simulink model "OpAmpOpenLoop"  (R2021b)
settings: Solver=VariableStepAuto  StartTime=0.0  StopTime=inf  MaxStep=1e-4  RelTol=1e-3
libraries: fl_lib x6, nesl_utility x4, ee_lib x1
settings Model: PacingRate=0.010000  Creator=Work  LastModifiedBy=Work

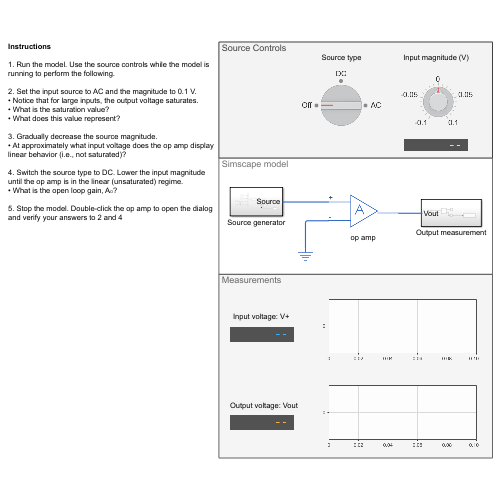
[thumbnail: Simulink's stored preview of the top-level diagram]
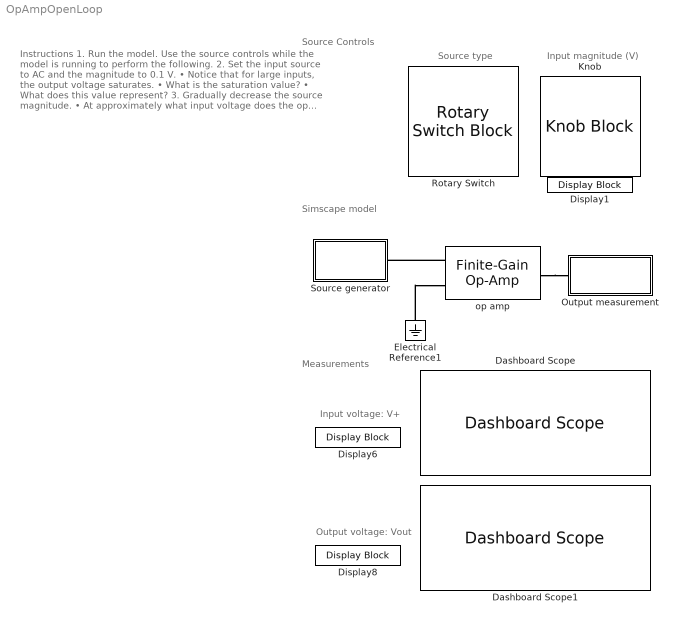
== system OpAmpOpenLoop ==
  note: Input magnitude (V)
  note: Source type
  note: Instructions
      |
      | 1. Run the model. Use the source controls while the model is running to perform the following.
      |
      | 2. Set the input source to AC and the magnitude to 0.1 V.
      | • Notice that for large inputs, the output voltage saturates.
      | • What is the saturation value?
      | • What does this value represent?
      |
      | 3. Gradually decrease the source magnitude.
      | • At approximately what input voltage does the op amp display linear behavior (i.e., not saturated)?
      |
      | 4. Switch the source type to DC. Lower the input magnitude until the op amp is in the linear (unsaturated) regime.
      | • What is the open loop gain, A O ?
      |
      | 5. Stop the model. Double-click the op amp to open the dialog and verify your answers to 2 and 4
  note: Source Controls
  note: Measurements
  note: Simscape model
  note: Input voltage: V+
  note: Output voltage: Vout
  Dashboard Scope : DashboardScope  TimeSpan=0.10000000000000001  Ymin=-0.15  Ymax=0.15  ScaleAtStop=off  UpdateMode=Scroll
  Dashboard Scope1 : DashboardScope  TimeSpan=0.10000000000000001  Ymin=-16  Ymax=16  ScaleAtStop=off  UpdateMode=Scroll
  Display1 : DisplayBlock  LabelPosition=Hide  Format=Custom  Alignment=Right  Transparency=1  FormatString=%0.4f
  Display6 : DisplayBlock  LabelPosition=Hide  Format=Custom  Alignment=Right  Transparency=1  FormatString=%0.4f
  Display8 : DisplayBlock  LabelPosition=Hide  Format=Custom  Alignment=Right  Transparency=1  FormatString=%0.4f
  Electrical Reference1 : fl_lib/Electrical/Electrical Elements/Electrical Reference
  Knob : KnobBlock  LabelPosition=Hide  ScaleMin=-0.1  ScaleMax=0.1  TickInterval=0.05
  Output measurement : Subsystem
  Rotary Switch : RotarySwitchBlock  LabelPosition=Hide
      settings: Values={{'Off', 'DC', 'AC'}, [0 1 2]}
  Source generator : Subsystem
  op amp : ee_lib/Integrated Circuits/Finite-Gain Op-Amp  A=2e3  Rin=1e6 Ohm  Rout=100 Ohm  Vmin=-15 V  Vmax=15 V  noise_mode=0  v_noise=30e-9 V/Hz^(1/2)  noise_prm=1  i_noise=0.5e-12 A/Hz^(1/2)  ip_noise=0.5e-12 A/Hz^(1/2)  in_noise=0.5e-12 A/Hz^(1/2)  sample_time=1e-3 s  repeatability=1  auto_seed_v=1041471841  auto_seed_ip=230873357  auto_seed_in=1897181789  user_seed_v=0  user_seed_ip=0  user_seed_in=0
      settings: SourceProductBaseCode=PS  InternalSimscapePortConfiguration="{\"Bottom\":[],\"Left\":[{\"id\":\"p\",\"label\":\"+\",\"type\":\"foundation.electrical.electrical\"},{\"id\":\"n\",\"label\":\"-\",\"type\":\"foundation.electrical.electrical\"}],\"Right\":[{\"id\":\"out\",\"label\":\"\",\"type\":\"foundation.electrical.electrical\"}],\"Top\":[]}"
  connections:
  Electrical Reference1/LConn1 -- op amp/LConn2
  op amp/LConn1 -- Source generator/RConn1
  op amp/RConn1 -- Output measurement/LConn1

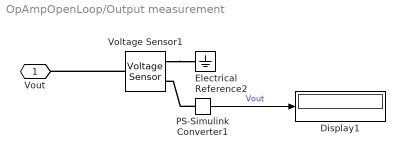
== system OpAmpOpenLoop/Output measurement ==
  Display1 : Display
  Electrical Reference2 : fl_lib/Electrical/Electrical Elements/Electrical Reference
  PS-Simulink Converter1 : nesl_utility/PS-Simulink Converter  PhysicalDomain=network_engine_domain  SubClassName=ps_output  LeftPortType=input  RightPortType=output  PseudoPeriodic=off  Frequencies=[]  Unit=inherit  AffineConversion=off
      settings: SourceProductBaseCode=PW,SS
  Voltage Sensor1 : fl_lib/Electrical/Electrical Sensors/Voltage Sensor
  Vout : PMIOPort  Side=Left
  wires:
  PS-Simulink Converter1/1 -> Display1/1  "Vout"
  connections:
  Voltage Sensor1/LConn1 -- Vout/RConn1
  Voltage Sensor1/RConn2 -- Electrical Reference2/LConn1
  PS-Simulink Converter1/LConn1 -- Voltage Sensor1/RConn1

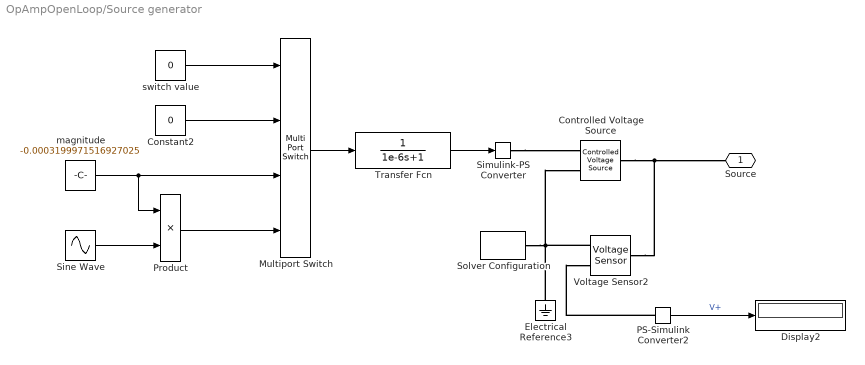
== system OpAmpOpenLoop/Source generator ==
  Constant2 : Constant  Value=0
  Controlled Voltage Source : fl_lib/Electrical/Electrical Sources/Controlled Voltage Source
  Display2 : Display
  Electrical Reference3 : fl_lib/Electrical/Electrical Elements/Electrical Reference
  Multiport Switch : MultiPortSwitch  DataPortOrder=Zero-based contiguous  zeroidx=on
  PS-Simulink Converter2 : nesl_utility/PS-Simulink Converter  PhysicalDomain=network_engine_domain  SubClassName=ps_output  LeftPortType=input  RightPortType=output  PseudoPeriodic=off  Frequencies=[]  Unit=inherit  AffineConversion=off
      settings: SourceProductBaseCode=PW,SS
  Product : Product
  Simulink-PS Converter : nesl_utility/Simulink-PS Converter  PhysicalDomain=network_engine_domain  SubClassName=ps_input  LeftPortType=input  RightPortType=output  PseudoPeriodic=off  Frequencies=[]  NoiseDistribution=none  NoiseParameters=[]  Unit=1  AffineConversion=off  FilteringAndDerivatives=provide  SimscapeFilterOrder=1  InputFilterTimeConstant=0.001  UdotUserProvided=0
      settings: SourceProductBaseCode=PW,SS
  Sine Wave : Sin  Frequency=2*pi*60  SampleTime=0
  Solver Configuration : nesl_utility/Solver Configuration  PhysicalDomain=network_engine_domain  SubClassName=solver  LeftPortType=input  RightPortType=generic  Tones=[]  Harmonics=[]  SimulateNoise=off  Profile=off  UseLocalSampling=off  EnableSwitchedLinearOptims=on  FrequencyDomain=off  UseCCode=off  RelTol=0.001  AbsTol=1e-06  MinStep=1e-09  ToWorkspace=off  RevertToSquareIcSolve=off  NumHomotopyIterations=100  PhasorMode=off  PhasorModeNumHarmonics=1  DoDC=off  ResidualTolerance=1e-09  UseLocalSolver=off  LocalSolverChoice=NE_BACKWARD_EULER_ADVANCER  LocalSolverSampleTime=0.001  DoFixedCost=off  MaxNonlinIter=3  MaxModeIter=2  ComputeImpulses=off  ImpulseIterations=2  LinearAlgebra=auto  EquationFormulation=NE_TIME_EF  DelaysMemoryBudget=1024  AutomaticFiltering=on  FilteringTimeConstant=0.001  PartitionStorageMethod=AS_NEEDED  PartitionMemoryBudget=1024  PartitionMethod=ROBUST
      settings: SourceProductBaseCode=PW,SS
  Transfer Fcn : TransferFcn  Denominator=[1e-6 1]
  Voltage Sensor2 : fl_lib/Electrical/Electrical Sensors/Voltage Sensor
  magnitude : Constant  Value=-0.0003199971516927025
  switch value : Constant  Value=0
  Source : PMIOPort  Side=Right
  wires:
  PS-Simulink Converter2/1 -> Display2/1  "V+"
  Sine Wave/1 -> Product/2
  magnitude/1 -> Multiport Switch/3, Product/1
  Product/1 -> Multiport Switch/4
  Multiport Switch/1 -> Transfer Fcn/1
  switch value/1 -> Multiport Switch/1
  Constant2/1 -> Multiport Switch/2
  Transfer Fcn/1 -> Simulink-PS Converter/1
  connections:
  Electrical Reference3/LConn1 -- Solver Configuration/RConn1 -- Voltage Sensor2/RConn2 -- Controlled Voltage Source/RConn2
  Controlled Voltage Source/LConn1 -- Voltage Sensor2/LConn1 -- Source/RConn1
  PS-Simulink Converter2/LConn1 -- Voltage Sensor2/RConn1
  Simulink-PS Converter/RConn1 -- Controlled Voltage Source/RConn1
